simulink model "FiltroV1"  (R2024b)
settings: Solver=VariableStepAuto  StartTime=0.0  StopTime=inf  RelTol=1e-3
libraries: dspfdesign x5, dspsnks4 x1, dspvision x1
settings Model: Creator=fredy  LastModifiedBy=fredy

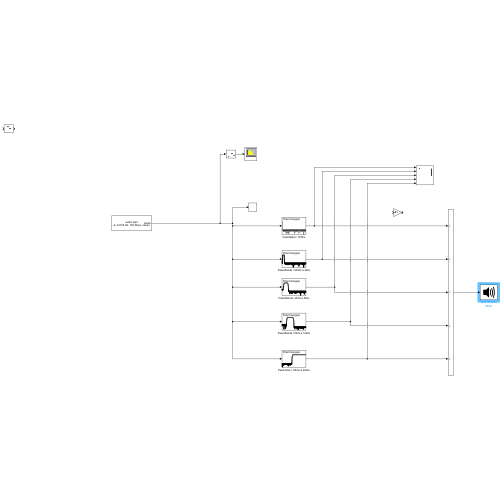
[thumbnail: Simulink's stored preview of the top-level diagram]
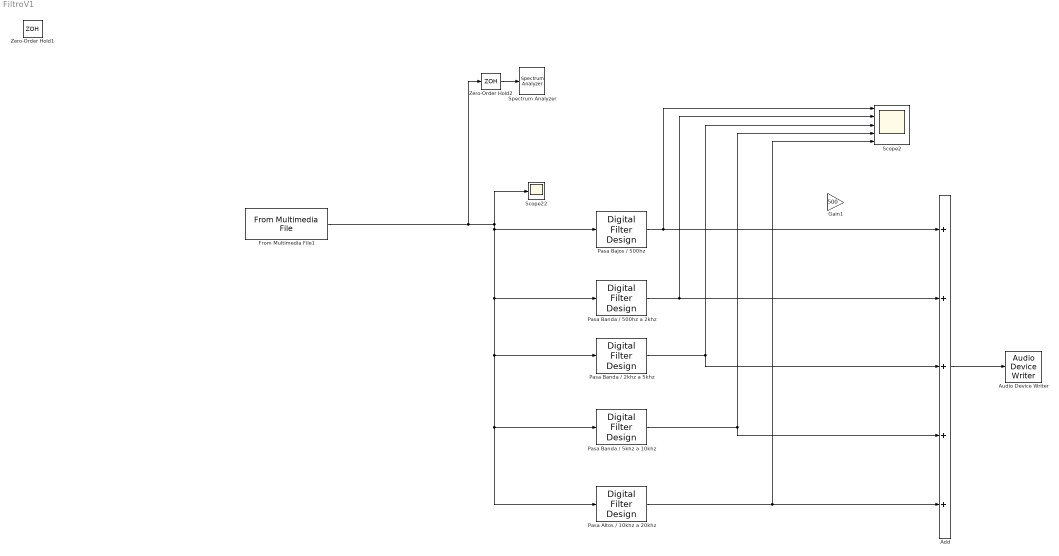
== system FiltroV1 ==
  Add : Sum  Inputs=+++++
  Audio Device Writer : dspsnks4/Audio Device Writer  Driver=DirectSound  Device=Default  InheritSampleRate=on  SampleRate=44100  BitDepth=16-bit integer  BufferSize=4096  NumBuffers=10  DefaultOutputChannelMapping=on  OutputChannelMapping=1:2  OutputNumUnderrunSamples=off  DriverIdx=1  DeviceWarnFlag=''
  From Multimedia File1 : dspvision/From Multimedia File  inputFilename=D:\Datos Fredy\Programacion\Matlab\Filtros\audio.mp3  readRange=[1 Inf]  loop=on  numPlays=inf  outputStreams=Audio only  videoDataType=single  audioDataType=single  inheritSampleTime=on  userDefinedSampleTime=1/30  noAudioOutput=off  isIntensityVideo=off  fourcc=RGB  colorVideoFormat=Separate color signals  outputEOF=off  dataOrg=Column-major  audioFrameSize=1  computeAudioFrameSize=off  outSamplingMode=Sample based
      settings: LibrarySourceBlock=audiosources/From Multimedia File
  Gain1 : Gain  Gain=500
  Pasa Altos / 10khz a 20khz : dspfdesign/Digital Filter Design  mwdsp_browser_bugfix_var=off
  Pasa Bajos / 500hz : dspfdesign/Digital Filter Design  mwdsp_browser_bugfix_var=off
  Pasa Banda / 2khz a 5khz : dspfdesign/Digital Filter Design  mwdsp_browser_bugfix_var=off
  Pasa Banda / 500hz a 2khz : dspfdesign/Digital Filter Design  mwdsp_browser_bugfix_var=off
  Pasa Banda / 5khz a 10khz : dspfdesign/Digital Filter Design  mwdsp_browser_bugfix_var=off
  Scope2 : Scope  NumInputPorts=5
  Scope22 : Scope
  Spectrum Analyzer : SpectrumAnalyzer  WindowPosition=[345.000000,488.000000,1132.000000,626.000000,]  ScopeFrameLocation=window  SampleRate=44.1e3  PlotAsTwoSidedSpectrum=off  FrequencyScale=Log  WindowInvariantSamplesPerUpdate=on  FrequencySpan=Start and stop frequencies  StartFrequency=20  YLimits=[-53.56074807,2.29453736]  SelectedToolstripTab=spectrumAnalyzerToolstrip.estimationTab
  Zero-Order Hold1 : ZeroOrderHold  SampleTime=0.0001
  Zero-Order Hold2 : ZeroOrderHold  SampleTime=0.0001
  wires:
  From Multimedia File1/1 -> Zero-Order Hold2/1, Pasa Banda / 500hz a 2khz/1, Pasa Banda / 2khz a 5khz/1, Pasa Altos / 10khz a 20khz/1, Pasa Banda / 5khz a 10khz/1, Pasa Bajos / 500hz/1, Scope22/1
  Zero-Order Hold2/1 -> Spectrum Analyzer/1
  Pasa Banda / 2khz a 5khz/1 -> Add/3, Scope2/3
  Pasa Banda / 5khz a 10khz/1 -> Add/4, Scope2/4
  Pasa Altos / 10khz a 20khz/1 -> Add/5, Scope2/5
  Pasa Banda / 500hz a 2khz/1 -> Add/2, Scope2/2
  Pasa Bajos / 500hz/1 -> Add/1, Scope2/1
  Add/1 -> Audio Device Writer/1
